simulink model "task4c_simulink"  (R2019b)
settings: Solver=VariableStepAuto  StartTime=0.0  StopTime=10.0  RelTol=1e-3
values from neighbouring files (symbols this model uses):
  A = [   -z m m n ... (first row only)    [det44.m]    (also in task1b.m = [1 1 1 0 0 0; task4c.m = [0 1; 0 0])
  B = [0; 1]    [task4c.m]
  C = eye(2)    [task4c.m]
  D = [1500; 2000; 1000]    [task1a.m]    (also in task4c.m = [0; 0])
  x0 = -10    [task4c.m]
undefined symbols (not defined in the file or in its folder): K
settings Model: Creator=Zac  LastModifiedBy=Zac

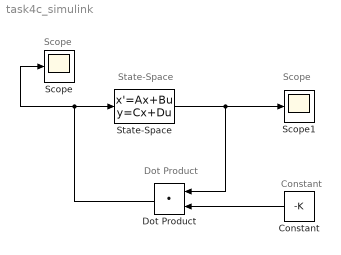
== system task4c_simulink ==
  note: State-Space
  note: Scope
  note: Constant
  note: Dot Product
  note: Scope
  Constant : Constant  Value=-K
  Dot Product : DotProduct  InputSameDT=on  OutDataTypeStr=Inherit: Inherit via internal rule
  Scope : Scope
  Scope1 : Scope
  State-Space : StateSpace  A=A  B=B  C=C  D=D  InitialCondition=x0
  wires:
  Dot Product/1 -> State-Space/1, Scope/1
  State-Space/1 -> Dot Product/1, Scope1/1
  Constant/1 -> Dot Product/2
